simulink model "SF018A_EotProtn"  (R2013b)
settings: Solver=FixedStepDiscrete  SolverMode=SingleTasking  StartTime=0.0  StopTime=0.002  FixedStep=.002  RelTol=1e-3
undefined symbols (not defined in the file): ALLSPDDAMPG_CNT_U08, ALLSPDGAIN_CNT_U08, ARCHGLBPRM_2MILLISEC_SEC_F32, DISTLPFILFRQ_HZ_F32, EOTDAMPGLOLIM_MOTNWTMTR_F32, EOTGAINHILIM_ULS_F32, EotProtnActvRegnBypMaxThd, EotProtnDampgSlew, EotProtnDampgVehSpdTbl, EotProtnDeltaTqThd, EotProtnDftPosn, EotProtnEntrGainVehSpdTbl, EotProtnEntrGainX, EotProtnEntrStLpFilFrq, EotProtnExitDampgY, EotProtnExitStLpFilFrq, EotProtnHwAgGain, EotProtnHwAgMax, EotProtnHwAgMin, EotProtnHwDegDampgX, EotProtnMotSpdIncptSca, EotProtnMotSpdIncptX, EotProtnMotSpdIncptY, EotProtnMotVelGain, EotProtnNormDampgY, EotProtnPosnRampStep, EotProtnRackTrvlLimrAuthyThd, EotProtnRackTrvlLimrAuthyThdLimd, EotProtnRackTrvlLimrEna, EotProtnRackTrvlLimrRng, EotProtnRackTrvlLimrRngLimd, EotProtnRackTrvlLimrVehSpdThd, EotProtnRunEotVelImpctAndSoftEndStop, EotProtnSoftEndStopAuthyThd, EotProtnSoftEndStopEna, EotProtnSoftEndStopVehSpdThd, FIRSTPTDAMPG_CNT_U08, LASTPTGAIN_CNT_U08, SOFTENDSTOPSTDI_CNT_U08, SOFTENDSTOPSTENTR_CNT_U08, SOFTENDSTOPSTEXIT_CNT_U08, SOFTENDSTOPSTNORM_CNT_U08, SYSGLBPRM_MOTTQCMDHILIM_MOTNWTMTR_F32, ZEROMOTTQCMD_MOTNWTMTR_F32
libraries: NxtrAbslt x16, FloatToFixd x14, FixdToFloat x6, Fil x5, NxtrLim x5, simulink x4, NxtrMax x4, LnrIntrpnDyn x3, NxtrSign x2, BilnrIntrpnMplXDyn x2, BilnrIntrpnMplX x1, LnrIntrpn x1
(part 3 of 5)

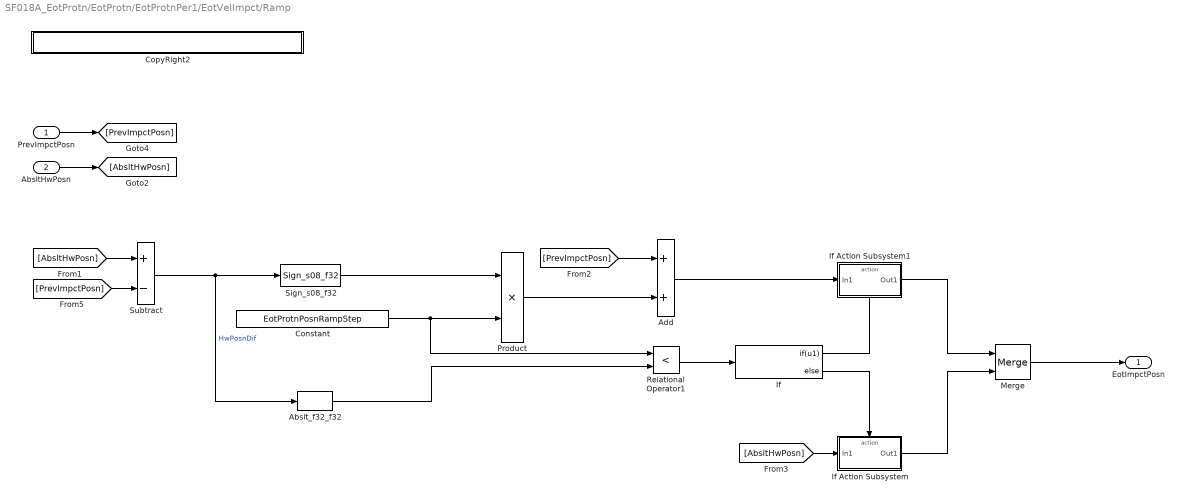
== system SF018A_EotProtn/EotProtn/EotProtnPer1/EotVelImpct/Ramp ==
  PrevImpctPosn : Inport
  AbsltHwPosn : Inport  Port=2
  Abslt_f32_f32 : NxtrAbslt/Abslt_f32_f32  RequirementInfo={'linktype_rmi_doors' '0000ba56 (/E-STEER Core/SubSystem Specifications/Application Functions/SF018A End-of-Travel Actuator Management- EOT Impact and Soft Stops)' '#SF018A_99' 'true' 'REQ: SF018A_99' '' } %GIDa_1abceffa_5429_43f7_acf2_7bb66654749d  SFunctionSpec=single y1 = Abslt_f32_f32(single u1)
      settings: AttributesFormatString=%<Name>
  Add : Sum  RequirementInfo={'linktype_rmi_doors' '0000ba56 (/E-STEER Core/SubSystem Specifications/Application Functions/SF018A End-of-Travel Actuator Management- EOT Impact and Soft Stops)' '#SF018A_99' 'true' 'REQ: SF018A_99' '' } %GIDa_4b3b0817_279b_45d5_a7ff_759bd2d41568
  Constant : Constant  RequirementInfo={'linktype_rmi_doors' '0000ba56 (/E-STEER Core/SubSystem Specifications/Application Functions/SF018A End-of-Travel Actuator Management- EOT Impact and Soft Stops)' '#SF018A_99' 'true' 'REQ: SF018A_99' '' } %GIDa_f7bca0cc_e413_4645_ac8d_d71262a020ac  Value=EotProtnPosnRampStep
  CopyRight2 : Subsystem  Description=|  mask(Copyright Information){none=on}
      | Copyright info block.                                               
      |                                                                     
      | Place copyright information at the top of every subsystem in design.
      mask prompts: none "No parameters"
      mask help: Place copyright information at the top of every subsystem in design.
      mask Display:
      | NxtrConf = 'Nexteer Confidential';
      | 
      | sys = bdroot; %handle for the current model ("system")
      | first = get_param(sys,'Created');
      | if(isempty(first))
      |     first = datestr(now,'yyyy');
      | else
      |     first = first(end-3:end);  %year is last four digits
      | end
      | 
      | last = get_param(sys,'LastModifiedDate');
      | if isempty(last)
      |     last = datestr(now,'yyyy');
      | else
      |     last = last(end-3:end);
      | end
      | 
      | if strcmp(first,last)
      |     fprintf('%s -- Copyright %s Nexteer',NxtrConf,first)
      | else
      |     fprintf('%s -- %s%s- %s Nexteer',NxtrConf,char(169),first,last)
      | end
  If : If  RequirementInfo={'linktype_rmi_doors' '0000ba56 (/E-STEER Core/SubSystem Specifications/Application Functions/SF018A End-of-Travel Actuator Management- EOT Impact and Soft Stops)' '#SF018A_99' 'true' 'REQ: SF018A_99' '' } %GIDa_742bd3cd_f3a7_4580_9ac8_68cba2588316  IfExpression=u1
  If Action Subsystem : Subsystem  RequirementInfo={'linktype_rmi_doors' '0000ba56 (/E-STEER Core/SubSystem Specifications/Application Functions/SF018A End-of-Travel Actuator Management- EOT Impact and Soft Stops)' '#SF018A_99' 'true' 'REQ: SF018A_99' '' } %GIDa_43f6df8e_6398_4b56_9d96_dcc88b087a3b  TreatAsAtomicUnit=on
  If Action Subsystem1 : Subsystem  RequirementInfo={'linktype_rmi_doors' '0000ba56 (/E-STEER Core/SubSystem Specifications/Application Functions/SF018A End-of-Travel Actuator Management- EOT Impact and Soft Stops)' '#SF018A_99' 'true' 'REQ: SF018A_99' '' } %GIDa_60fb960e_afb5_4503_a9d1_873d957e00f4  TreatAsAtomicUnit=on
  Merge : Merge  RequirementInfo={'linktype_rmi_doors' '0000ba56 (/E-STEER Core/SubSystem Specifications/Application Functions/SF018A End-of-Travel Actuator Management- EOT Impact and Soft Stops)' '#SF018A_99' 'true' 'REQ: SF018A_99' '' } %GIDa_980ed3f9_6cab_48af_a5f8_074a3afd95c0
  Product : Product  RequirementInfo={'linktype_rmi_doors' '0000ba56 (/E-STEER Core/SubSystem Specifications/Application Functions/SF018A End-of-Travel Actuator Management- EOT Impact and Soft Stops)' '#SF018A_99' 'true' 'REQ: SF018A_99' '' } %GIDa_1965b7b1_3372_4a34_81de_e822cfa0f36c  RndMeth=Zero
  Relational Operator1 : RelationalOperator  RequirementInfo={'linktype_rmi_doors' '0000ba56 (/E-STEER Core/SubSystem Specifications/Application Functions/SF018A End-of-Travel Actuator Management- EOT Impact and Soft Stops)' '#SF018A_99' 'true' 'REQ: SF018A_99' '' } %GIDa_2c3f3792_848e_4354_937e_e14b12a6658e  Operator=<  OutDataTypeStr=boolean
  Sign_s08_f32 : NxtrSign/Sign_s08_f32  RequirementInfo={'linktype_rmi_doors' '0000ba56 (/E-STEER Core/SubSystem Specifications/Application Functions/SF018A End-of-Travel Actuator Management- EOT Impact and Soft Stops)' '#SF018A_99' 'true' 'REQ: SF018A_99' '' } %GIDa_dea15310_ec68_42a1_8b11_5567d207a828  SFunctionSpec=int8 y1 = Sign_s08_f32(single u1)
  Subtract : Sum  RequirementInfo={'linktype_rmi_doors' '0000ba56 (/E-STEER Core/SubSystem Specifications/Application Functions/SF018A End-of-Travel Actuator Management- EOT Impact and Soft Stops)' '#SF018A_99' 'true' 'REQ: SF018A_99' '' } %GIDa_d23a2f2b_f22f_4421_a8b2_6f0d87dd44f6  Inputs=+-
  EotImpctPosn : Outport
  wires:
  Relational Operator1/1 -> If/1
  If/1 -> If Action Subsystem1/Action
  If/2 -> If Action Subsystem/Action
  If Action Subsystem/1(Out1) -> Merge/2
  If Action Subsystem1/1(Out1) -> Merge/1
  Add/1 -> If Action Subsystem1/1(In1)
  [AbsltHwPosn] -> If Action Subsystem/1(In1)
  Merge/1 -> EotImpctPosn/1
  [PrevImpctPosn] -> Add/1
  Product/1 -> Add/2
  Abslt_f32_f32/1 -> Relational Operator1/2
  Sign_s08_f32/1 -> Product/1
  Constant/1 -> Product/2, Relational Operator1/1
  Subtract/1 -> Sign_s08_f32/1, Abslt_f32_f32/1  "HwPosnDif"
  [PrevImpctPosn] -> Subtract/2
  [AbsltHwPosn] -> Subtract/1
  AbsltHwPosn/1 -> [AbsltHwPosn]
  PrevImpctPosn/1 -> [PrevImpctPosn]

== system SF018A_EotProtn/EotProtn/EotProtnPer1/If Action Subsystem/CopyRight2 ==

== system SF018A_EotProtn/EotProtn/EotProtnPer1/If Action Subsystem5/CopyRight2 ==

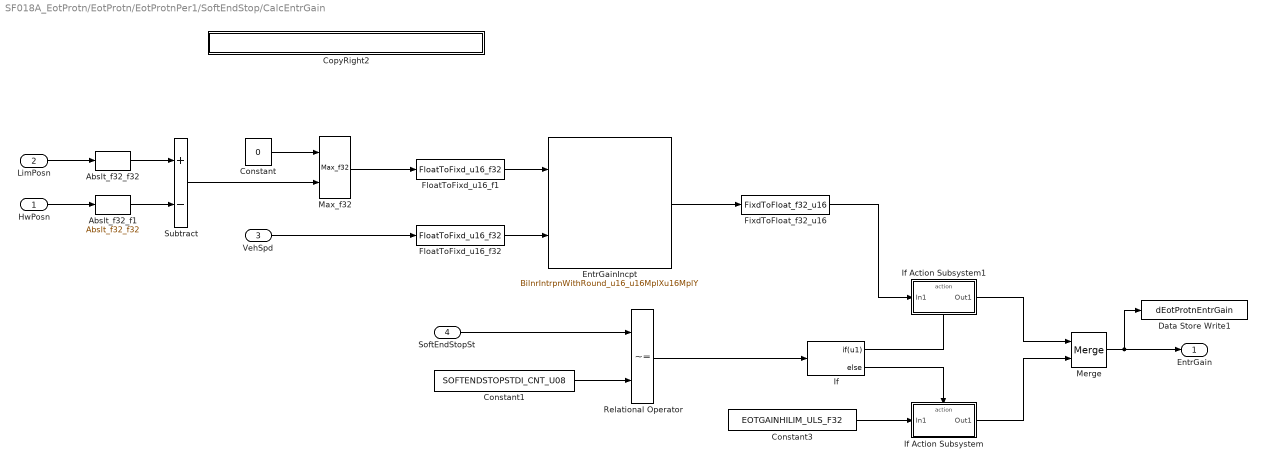
== system SF018A_EotProtn/EotProtn/EotProtnPer1/SoftEndStop/CalcEntrGain ==
  HwPosn : Inport
  LimPosn : Inport  Port=2
  VehSpd : Inport  Port=3
  SoftEndStopSt : Inport  Port=4
  Abslt_f32_f1 : NxtrAbslt/Abslt_f32_f32  SFunctionSpec=single y1 = Abslt_f32_f32(single u1)
      settings: AttributesFormatString=%<Name>
  Abslt_f32_f32 : NxtrAbslt/Abslt_f32_f32  SFunctionSpec=single y1 = Abslt_f32_f32(single u1)
      settings: AttributesFormatString=%<Name>
  Constant : Constant  Value=0  OutDataTypeStr=single
  Constant1 : Constant  Value=SOFTENDSTOPSTDI_CNT_U08
  Constant3 : Constant  RequirementInfo={'linktype_rmi_doors' '0000ba56 (/E-STEER Core/SubSystem Specifications/Application Functions/SF018A End-of-Travel Actuator Management- EOT Impact and Soft Stops)' '#SF018A_110' 'true' 'REQ: SF018A_110' '' } %GIDa_44744990_5e4e_4c9c_97f2_54307b70273a  Value=EOTGAINHILIM_ULS_F32
  CopyRight2 : Subsystem  Description=|  mask(Copyright Information){none=on}
      | Copyright info block.                                               
      |                                                                     
      | Place copyright information at the top of every subsystem in design.
      mask prompts: none "No parameters"
      mask help: Place copyright information at the top of every subsystem in design.
      mask Display:
      | NxtrConf = 'Nexteer Confidential';
      | 
      | sys = bdroot; %handle for the current model ("system")
      | first = get_param(sys,'Created');
      | if(isempty(first))
      |     first = datestr(now,'yyyy');
      | else
      |     first = first(end-3:end);  %year is last four digits
      | end
      | 
      | last = get_param(sys,'LastModifiedDate');
      | if isempty(last)
      |     last = datestr(now,'yyyy');
      | else
      |     last = last(end-3:end);
      | end
      | 
      | if strcmp(first,last)
      |     fprintf('%s -- Copyright %s Nexteer',NxtrConf,first)
      | else
      |     fprintf('%s -- %s%s- %s Nexteer',NxtrConf,char(169),first,last)
      | end
  Data Store Write1 : DataStoreWrite  DataStoreName=dEotProtnEntrGain
  EntrGainIncpt : BilnrIntrpnMplX/BilnrIntrpnWithRound_u16_u16MplXu16MplY  RequirementInfo={'linktype_rmi_doors' '0000ba56 (/E-STEER Core/SubSystem Specifications/Application Functions/SF018A End-of-Travel Actuator Management- EOT Impact and Soft Stops)' '#SF018A_106' 'true' 'REQ: SF018A_106' '' } %GIDa_4fff3482_45f7_455a_b7ca_7ca531bddd7e  MplXTbl=EotProtnEntrGainX  MplYTbl=EotProtnEntrGainY  BilnrSelnTbl=EotProtnEntrGainVehSpdTbl
      settings: AttributesFormatString=Bilnr ( u16MplX , u16MplY )
  FixdToFloat_f32_u16 : FixdToFloat/FixdToFloat_f32_u16  Param1=15
  FloatToFixd_u16_f1 : FloatToFixd/FloatToFixd_u16_f32  Param1=4
  FloatToFixd_u16_f32 : FloatToFixd/FloatToFixd_u16_f32  Param1=7
  If : If  RequirementInfo={'linktype_rmi_doors' '0000ba56 (/E-STEER Core/SubSystem Specifications/Application Functions/SF018A End-of-Travel Actuator Management- EOT Impact and Soft Stops)' '#SF018A_110' 'true' 'REQ: SF018A_110' '' } %GIDa_9ba4167e_05f8_43ad_8506_1cfb529838b9  IfExpression=u1
  If Action Subsystem : Subsystem  RequirementInfo={'linktype_rmi_doors' '0000ba56 (/E-STEER Core/SubSystem Specifications/Application Functions/SF018A End-of-Travel Actuator Management- EOT Impact and Soft Stops)' '#SF018A_110' 'true' 'REQ: SF018A_110' '' } %GIDa_2636f089_91d8_4ceb_8b94_5c1d30901327  TreatAsAtomicUnit=on
  If Action Subsystem1 : Subsystem  RequirementInfo={'linktype_rmi_doors' '0000ba56 (/E-STEER Core/SubSystem Specifications/Application Functions/SF018A End-of-Travel Actuator Management- EOT Impact and Soft Stops)' '#SF018A_110' 'true' 'REQ: SF018A_110' '' } %GIDa_4dab6c91_13d9_4980_84a7_ab8b61b230ac  TreatAsAtomicUnit=on
  Max_f32 : NxtrMax/Max_f32  SFunctionSpec=single y1 = Max_f32(single u1, single u2)
      settings: AttributesFormatString=%<Name>
  Merge : Merge  RequirementInfo={'linktype_rmi_doors' '0000ba56 (/E-STEER Core/SubSystem Specifications/Application Functions/SF018A End-of-Travel Actuator Management- EOT Impact and Soft Stops)' '#SF018A_110' 'true' 'REQ: SF018A_110' '' } %GIDa_f387e512_66e3_47bc_bfbf_7513709a11a9
  Relational Operator : RelationalOperator  RequirementInfo={'linktype_rmi_doors' '0000ba56 (/E-STEER Core/SubSystem Specifications/Application Functions/SF018A End-of-Travel Actuator Management- EOT Impact and Soft Stops)' '#SF018A_110' 'true' 'REQ: SF018A_110' '' } %GIDa_a3a9fdec_6549_4f75_9399_aedfe2c4c451  Operator=~=  OutDataTypeStr=boolean
  Subtract : Sum  RequirementInfo={'linktype_rmi_doors' '0000ba56 (/E-STEER Core/SubSystem Specifications/Application Functions/SF018A End-of-Travel Actuator Management- EOT Impact and Soft Stops)' '#SF018A_106' 'true' 'REQ: SF018A_106' '' } %GIDa_7ecf2b4b_fe31_40cc_9806_1ed7231da289  Inputs=+-
  EntrGain : Outport
  wires:
  EntrGainIncpt/1 -> FixdToFloat_f32_u16/1
  FloatToFixd_u16_f1/1 -> EntrGainIncpt/1
  Relational Operator/1 -> If/1
  FixdToFloat_f32_u16/1 -> If Action Subsystem1/1(In1)
  Max_f32/1 -> FloatToFixd_u16_f1/1
  Constant/1 -> Max_f32/1
  Constant1/1 -> Relational Operator/2
  Merge/1 -> EntrGain/1, Data Store Write1/1
  Constant3/1 -> If Action Subsystem/1(In1)
  SoftEndStopSt/1 -> Relational Operator/1
  If/1 -> If Action Subsystem1/Action
  If/2 -> If Action Subsystem/Action
  If Action Subsystem/1(Out1) -> Merge/2
  If Action Subsystem1/1(Out1) -> Merge/1
  FloatToFixd_u16_f32/1 -> EntrGainIncpt/2
  VehSpd/1 -> FloatToFixd_u16_f32/1
  Subtract/1 -> Max_f32/2
  Abslt_f32_f1/1 -> Subtract/2
  Abslt_f32_f32/1 -> Subtract/1
  LimPosn/1 -> Abslt_f32_f32/1
  HwPosn/1 -> Abslt_f32_f1/1

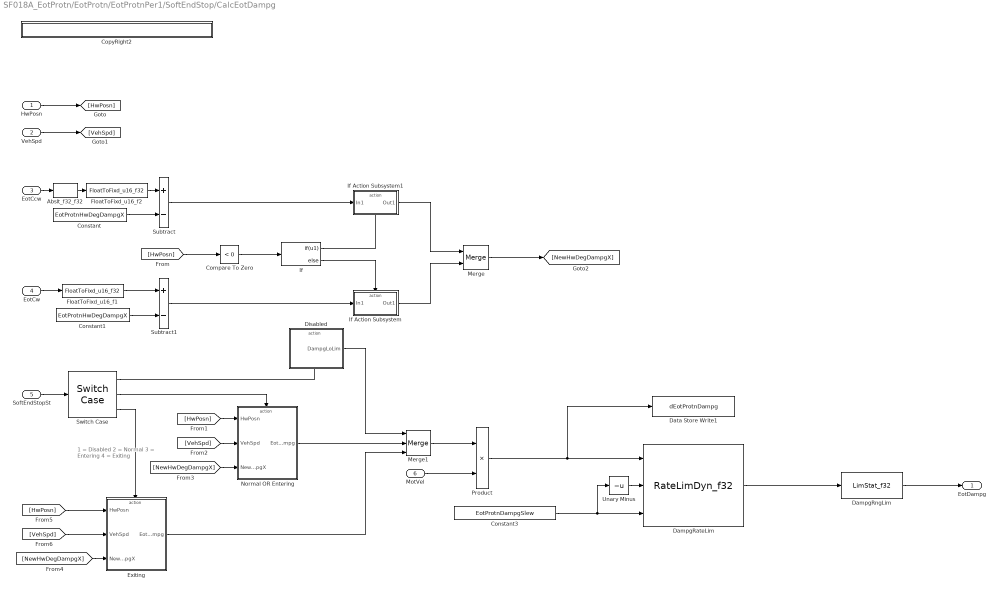
== system SF018A_EotProtn/EotProtn/EotProtnPer1/SoftEndStop/CalcEotDampg ==
  note: 1 = Disabled
      | 2 = Normal
      | 3 = Entering
      | 4 = Exiting
  HwPosn : Inport
  VehSpd : Inport  Port=2
  EotCcw : Inport  Port=3
  EotCw : Inport  Port=4
  SoftEndStopSt : Inport  Port=5
  MotVel : Inport  Port=6
  " Disabled" : Subsystem  RequirementInfo={'linktype_rmi_doors' '0000ba56 (/E-STEER Core/SubSystem Specifications/Application Functions/SF018A End-of-Travel Actuator Management- EOT Impact and Soft Stops)' '#SF018A_112' 'true' 'REQ: SF018A_112' '' } %GIDa_ecfa1b07_e2c5_474f_af19_fddfe94ef9e6
  " Exiting" : Subsystem  TreatAsAtomicUnit=on
  " Normal OR Entering" : Subsystem  TreatAsAtomicUnit=on
  Abslt_f32_f32 : NxtrAbslt/Abslt_f32_f32  SFunctionSpec=single y1 = Abslt_f32_f32(single u1)
      settings: AttributesFormatString=%<Name>
  Compare To Zero : simulink/Logic and Bit Operations/Compare To Zero  RequirementInfo={'linktype_rmi_doors' '0000ba56 (/E-STEER Core/SubSystem Specifications/Application Functions/SF018A End-of-Travel Actuator Management- EOT Impact and Soft Stops)' '#SF018A_112' 'true' 'REQ: SF018A_112' '' } %GIDa_9be31a75_f41f_436f_9025_b1c96be2af0a  relop=<  OutDataTypeStr=boolean
  Constant : Constant  RequirementInfo={'linktype_rmi_doors' '0000ba56 (/E-STEER Core/SubSystem Specifications/Application Functions/SF018A End-of-Travel Actuator Management- EOT Impact and Soft Stops)' '#SF018A_112' 'true' 'REQ: SF018A_112' '' } %GIDa_dbcb604d_2f24_40f5_8854_e760e508102d  Value=EotProtnHwDegDampgX
  Constant1 : Constant  RequirementInfo={'linktype_rmi_doors' '0000ba56 (/E-STEER Core/SubSystem Specifications/Application Functions/SF018A End-of-Travel Actuator Management- EOT Impact and Soft Stops)' '#SF018A_112' 'true' 'REQ: SF018A_112' '' } %GIDa_c66114bb_2673_4ad0_b25b_e6b85f1e3550  Value=EotProtnHwDegDampgX
  Constant3 : Constant  RequirementInfo={'linktype_rmi_doors' '0000ba56 (/E-STEER Core/SubSystem Specifications/Application Functions/SF018A End-of-Travel Actuator Management- EOT Impact and Soft Stops)' '#SF018A_107' 'true' 'REQ: SF018A_107' '' ; 'linktype_rmi_doors' '0000ba56 (/E-STEER Core/SubSystem Specifications/Application Functions/SF018A End-of-Travel Actuator Management- EOT Impact and Soft Stops)' '#SF018A_108' 'true' 'REQ: SF018A_108' '' } %GIDa_b144d1b2_0f77_499c_8b78_f2421302eedf  Value=EotProtnDampgSlew
  CopyRight2 : Subsystem  Description=|  mask(Copyright Information){none=on}
      | Copyright info block.                                               
      |                                                                     
      | Place copyright information at the top of every subsystem in design.
      mask prompts: none "No parameters"
      mask help: Place copyright information at the top of every subsystem in design.
      mask Display:
      | NxtrConf = 'Nexteer Confidential';
      | 
      | sys = bdroot; %handle for the current model ("system")
      | first = get_param(sys,'Created');
      | if(isempty(first))
      |     first = datestr(now,'yyyy');
      | else
      |     first = first(end-3:end);  %year is last four digits
      | end
      | 
      | last = get_param(sys,'LastModifiedDate');
      | if isempty(last)
      |     last = datestr(now,'yyyy');
      | else
      |     last = last(end-3:end);
      | end
      | 
      | if strcmp(first,last)
      |     fprintf('%s -- Copyright %s Nexteer',NxtrConf,first)
      | else
      |     fprintf('%s -- %s%s- %s Nexteer',NxtrConf,char(169),first,last)
      | end
  DampgRateLim : NxtrLim/RateLimDyn_f32  RequirementInfo={'linktype_rmi_doors' '0000ba56 (/E-STEER Core/SubSystem Specifications/Application Functions/SF018A End-of-Travel Actuator Management- EOT Impact and Soft Stops)' '#SF018A_107' 'true' 'REQ: SF018A_107' '' ; 'linktype_rmi_doors' '0000ba56 (/E-STEER Core/SubSystem Specifications/Application Functions/SF018A End-of-Travel Actuator Management- EOT Impact and Soft Stops)' '#SF018A_108' 'true' 'REQ: SF018A_108' '' } %GIDa_7842721c_96f0_4555_8d64_95f51b59d9d7  StVar=PrevEotDampg  Ts=ARCHGLBPRM_2MILLISEC_SEC_F32
      link override Data Store Read: DataStoreName=PrevEotDampg
      link override Data Store Write: DataStoreName=PrevEotDampg
      settings: AttributesFormatString=StVar: %<StVar>
  DampgRngLim : NxtrLim/LimStat_f32  RequirementInfo={'linktype_rmi_doors' '0000ba56 (/E-STEER Core/SubSystem Specifications/Application Functions/SF018A End-of-Travel Actuator Management- EOT Impact and Soft Stops)' '#SF018A_113' 'true' 'REQ: SF018A_113' '' } %GIDa_f21829fe_30fb_47d7_986c_fd83414cd0bc  LoLim=SYSGLBPRM_MOTTQCMDLOLIM_MOTNWTMTR_F32  HiLim=SYSGLBPRM_MOTTQCMDHILIM_MOTNWTMTR_F32
      settings: AttributesFormatString=|
      | Low Limit: %<LoLim>
      | High Limit:%<HiLim>
  Data Store Write1 : DataStoreWrite  DataStoreName=dEotProtnDampg
  FloatToFixd_u16_f1 : FloatToFixd/FloatToFixd_u16_f32  Param1=4
  FloatToFixd_u16_f2 : FloatToFixd/FloatToFixd_u16_f32  Param1=4
  If : If  RequirementInfo={'linktype_rmi_doors' '0000ba56 (/E-STEER Core/SubSystem Specifications/Application Functions/SF018A End-of-Travel Actuator Management- EOT Impact and Soft Stops)' '#SF018A_112' 'true' 'REQ: SF018A_112' '' } %GIDa_80fe16f3_461b_464d_939e_d39adab0e653  IfExpression=u1
  If Action Subsystem : Subsystem  RequirementInfo={'linktype_rmi_doors' '0000ba56 (/E-STEER Core/SubSystem Specifications/Application Functions/SF018A End-of-Travel Actuator Management- EOT Impact and Soft Stops)' '#SF018A_112' 'true' 'REQ: SF018A_112' '' } %GIDa_e943b242_c41a_47ba_8233_2176091eed70  TreatAsAtomicUnit=on
  If Action Subsystem1 : Subsystem  RequirementInfo={'linktype_rmi_doors' '0000ba56 (/E-STEER Core/SubSystem Specifications/Application Functions/SF018A End-of-Travel Actuator Management- EOT Impact and Soft Stops)' '#SF018A_112' 'true' 'REQ: SF018A_112' '' } %GIDa_bde328e5_3b39_4d8b_939f_44ff43e1078d  TreatAsAtomicUnit=on
  Merge : Merge  RequirementInfo={'linktype_rmi_doors' '0000ba56 (/E-STEER Core/SubSystem Specifications/Application Functions/SF018A End-of-Travel Actuator Management- EOT Impact and Soft Stops)' '#SF018A_112' 'true' 'REQ: SF018A_112' '' } %GIDa_c1aa902f_1f6f_4629_beda_cf4686bd9346
  Merge1 : Merge  RequirementInfo={'linktype_rmi_doors' '0000ba56 (/E-STEER Core/SubSystem Specifications/Application Functions/SF018A End-of-Travel Actuator Management- EOT Impact and Soft Stops)' '#SF018A_112' 'true' 'REQ: SF018A_112' '' } %GIDa_e0e5e6ca_8c3a_4f1c_bb6f_ec62d627a8cd  Inputs=3
  Product : Product  RequirementInfo={'linktype_rmi_doors' '0000ba56 (/E-STEER Core/SubSystem Specifications/Application Functions/SF018A End-of-Travel Actuator Management- EOT Impact and Soft Stops)' '#SF018A_112' 'true' 'REQ: SF018A_112' '' } %GIDa_edec6862_a88c_4eda_8732_0ab8679f0f39  RndMeth=Zero
  Subtract : Sum  RequirementInfo={'linktype_rmi_doors' '0000ba56 (/E-STEER Core/SubSystem Specifications/Application Functions/SF018A End-of-Travel Actuator Management- EOT Impact and Soft Stops)' '#SF018A_112' 'true' 'REQ: SF018A_112' '' } %GIDa_fd2362af_1e36_467c_917a_9f3405f6ac8b  Inputs=+-
  Subtract1 : Sum  RequirementInfo={'linktype_rmi_doors' '0000ba56 (/E-STEER Core/SubSystem Specifications/Application Functions/SF018A End-of-Travel Actuator Management- EOT Impact and Soft Stops)' '#SF018A_112' 'true' 'REQ: SF018A_112' '' } %GIDa_c20c8d7b_5540_434b_b02f_ea8a96eddc7e  Inputs=+-
  Switch Case : SwitchCase  RequirementInfo={'linktype_rmi_doors' '0000ba56 (/E-STEER Core/SubSystem Specifications/Application Functions/SF018A End-of-Travel Actuator Management- EOT Impact and Soft Stops)' '#SF018A_112' 'true' 'REQ: SF018A_112' '' } %GIDa_87bdb368_40c5_441a_b972_d5c9fc169f63  CaseConditions={1,[2,3],4}  ShowDefaultCase=off
  Unary Minus : UnaryMinus  RequirementInfo={'linktype_rmi_doors' '0000ba56 (/E-STEER Core/SubSystem Specifications/Application Functions/SF018A End-of-Travel Actuator Management- EOT Impact and Soft Stops)' '#SF018A_107' 'true' 'REQ: SF018A_107' '' ; 'linktype_rmi_doors' '0000ba56 (/E-STEER Core/SubSystem Specifications/Application Functions/SF018A End-of-Travel Actuator Management- EOT Impact and Soft Stops)' '#SF018A_108' 'true' 'REQ: SF018A_108' '' } %GIDa_64f4e9aa_203f_4d05_a587_f31f06ac7c23
  EotDampg : Outport
  wires:
  DampgRngLim/1 -> EotDampg/1
  SoftEndStopSt/1 -> Switch Case/1
  Merge1/1 -> Product/1
  DampgRateLim/1 -> DampgRngLim/1
  Subtract/1 -> If Action Subsystem1/1(In1)
  Constant/1 -> Subtract/2
  [HwPosn] -> " Normal OR Entering"/1(HwPosn)
  Unary Minus/1 -> DampgRateLim/2
  Constant3/1 -> DampgRateLim/3, Unary Minus/1
  Product/1 -> DampgRateLim/1, Data Store Write1/1
  MotVel/1 -> Product/2
  " Exiting"/1(EotDampg) -> Merge1/3
  " Normal OR Entering"/1(EotDampg) -> Merge1/2
  " Disabled"/1(DampgLoLim) -> Merge1/1
  [VehSpd] -> " Exiting"/2(VehSpd)
  [HwPosn] -> " Exiting"/1(HwPosn)
  [NewHwDegDampgX] -> " Exiting"/3(NewHwDegDampgX)
  Switch Case/3 -> " Exiting"/Action
  [VehSpd] -> " Normal OR Entering"/2(VehSpd)
  [NewHwDegDampgX] -> " Normal OR Entering"/3(NewHwDegDampgX)
  Switch Case/2 -> " Normal OR Entering"/Action
  Switch Case/1 -> " Disabled"/Action
  Merge/1 -> [NewHwDegDampgX]
  Subtract1/1 -> If Action Subsystem/1(In1)
  Compare To Zero/1 -> If/1
  If/1 -> If Action Subsystem1/Action
  If/2 -> If Action Subsystem/Action
  If Action Subsystem/1(Out1) -> Merge/2
  If Action Subsystem1/1(Out1) -> Merge/1
  Constant1/1 -> Subtract1/2
  FloatToFixd_u16_f1/1 -> Subtract1/1
  EotCw/1 -> FloatToFixd_u16_f1/1
  [HwPosn] -> Compare To Zero/1
  FloatToFixd_u16_f2/1 -> Subtract/1
  EotCcw/1 -> Abslt_f32_f32/1
  VehSpd/1 -> [VehSpd]
  HwPosn/1 -> [HwPosn]
  Abslt_f32_f32/1 -> FloatToFixd_u16_f2/1

== system SF018A_EotProtn/EotProtn/EotProtnPer1/SoftEndStop/CalcEotGain ==
  note: 1 = Disabled
      | 2 = Normal
      | 3 = Entering
      | 4 = Exiting
  EntrGain : Inport
  SoftEndStopSt : Inport  Port=2
  ExitGain : Inport  Port=3
  " Disabled" : Subsystem  RequirementInfo={'linktype_rmi_doors' '0000ba56 (/E-STEER Core/SubSystem Specifications/Application Functions/SF018A End-of-Travel Actuator Management- EOT Impact and Soft Stops)' '#SF018A_110' 'true' 'REQ: SF018A_110' '' } %GIDa_08480493_e720_439d_8401_9a38b0039812
  " Exiting" : Subsystem
  Constant : Constant  RequirementInfo={'linktype_rmi_doors' '0000ba56 (/E-STEER Core/SubSystem Specifications/Application Functions/SF018A End-of-Travel Actuator Management- EOT Impact and Soft Stops)' '#SF018A_110' 'true' 'REQ: SF018A_110' '' } %GIDa_76f8a074_7de7_475c_bca0_9f449228cd27  Value=EOTGAINHILIM_ULS_F32
  CopyRight2 : Subsystem  Description=|  mask(Copyright Information){none=on}
      | Copyright info block.                                               
      |                                                                     
      | Place copyright information at the top of every subsystem in design.
      mask prompts: none "No parameters"
      mask help: Place copyright information at the top of every subsystem in design.
      mask Display:
      | NxtrConf = 'Nexteer Confidential';
      | 
      | sys = bdroot; %handle for the current model ("system")
      | first = get_param(sys,'Created');
      | if(isempty(first))
      |     first = datestr(now,'yyyy');
      | else
      |     first = first(end-3:end);  %year is last four digits
      | end
      | 
      | last = get_param(sys,'LastModifiedDate');
      | if isempty(last)
      |     last = datestr(now,'yyyy');
      | else
      |     last = last(end-3:end);
      | end
      | 
      | if strcmp(first,last)
      |     fprintf('%s -- Copyright %s Nexteer',NxtrConf,first)
      | else
      |     fprintf('%s -- %s%s- %s Nexteer',NxtrConf,char(169),first,last)
      | end
  Data Store Write1 : DataStoreWrite  DataStoreName=dEotProtnEotGain
  Entering or Normal : Subsystem
  Merge : Merge  Inputs=3
  Switch Case : SwitchCase  CaseConditions={1,4}
  EotGain : Outport
  wires:
  SoftEndStopSt/1 -> Switch Case/1
  " Disabled"/1(Out1) -> Merge/1
  Constant/1 -> " Disabled"/1(In1)
  Merge/1 -> EotGain/1, Data Store Write1/1
  EntrGain/1 -> Entering or Normal/1(In1)
  ExitGain/1 -> " Exiting"/1(In1)
  Entering or Normal/1(Out1) -> Merge/3
  " Exiting"/1(Out1) -> Merge/2
  Switch Case/3 -> Entering or Normal/Action
  Switch Case/2 -> " Exiting"/Action
  Switch Case/1 -> " Disabled"/Action

== system SF018A_EotProtn/EotProtn/EotProtnPer1/SoftEndStop/CalcExitGain ==
  HwTq : Inport
  HwPosn : Inport  Port=2
  PrevEotAssiSca : Inport  Port=3
  Abslt_f32_f32 : NxtrAbslt/Abslt_f32_f32  SFunctionSpec=single y1 = Abslt_f32_f32(single u1)
      settings: AttributesFormatString=%<Name>
  CopyRight2 : Subsystem  Description=|  mask(Copyright Information){none=on}
      | Copyright info block.                                               
      |                                                                     
      | Place copyright information at the top of every subsystem in design.
      mask prompts: none "No parameters"
      mask help: Place copyright information at the top of every subsystem in design.
      mask Display:
      | NxtrConf = 'Nexteer Confidential';
      | 
      | sys = bdroot; %handle for the current model ("system")
      | first = get_param(sys,'Created');
      | if(isempty(first))
      |     first = datestr(now,'yyyy');
      | else
      |     first = first(end-3:end);  %year is last four digits
      | end
      | 
      | last = get_param(sys,'LastModifiedDate');
      | if isempty(last)
      |     last = datestr(now,'yyyy');
      | else
      |     last = last(end-3:end);
      | end
      | 
      | if strcmp(first,last)
      |     fprintf('%s -- Copyright %s Nexteer',NxtrConf,first)
      | else
      |     fprintf('%s -- %s%s- %s Nexteer',NxtrConf,char(169),first,last)
      | end
  Data Store Write1 : DataStoreWrite  DataStoreName=dEotProtnExitGain
  FilLpUpdOutp : Fil/FilLpUpdOutp  StVar=HwTqLpFil
      settings: AttributesFormatString=StVar: %<StVar>
  FixdToFloat_f32_u16 : FixdToFloat/FixdToFloat_f32_u16  Param1=8
  FloatToFixd_u16_f32 : FloatToFixd/FloatToFixd_u16_f32  Param1=12
  Max_f32 : NxtrMax/Max_f32  RequirementInfo={'linktype_rmi_doors' '0000ba56 (/E-STEER Core/SubSystem Specifications/Application Functions/SF018A End-of-Travel Actuator Management- EOT Impact and Soft Stops)' '#SF018A_106' 'true' 'REQ: SF018A_106' '' } %GIDa_2332db26_7b5a_450a_9ed5_06682af17ddf  SFunctionSpec=single y1 = Max_f32(single u1, single u2)
      settings: AttributesFormatString=%<Name>
  Product : Product  RndMeth=Zero
  Sign_s08_f32 : NxtrSign/Sign_s08_f32  SFunctionSpec=int8 y1 = Sign_s08_f32(single u1)
  TqGainTbl : LnrIntrpn/LnrIntrpn_u16_u16VariXu16VariY  RequirementInfo={'linktype_rmi_doors' '0000ba56 (/E-STEER Core/SubSystem Specifications/Application Functions/SF018A End-of-Travel Actuator Management- EOT Impact and Soft Stops)' '#SF018A_106' 'true' 'REQ: SF018A_106' '' } %GIDa_1f060768_d7a3_4390_b9e3_be263574284b  XTbl=EotProtnHwTqScaX  YTbl=HWTQSCAY_ULS_U8P8
      settings: AttributesFormatString=Lnr ( u16VariX , u16VariY )
  ExitGain : Outport
  FildHwTq : Outport  Port=2
  wires:
  TqGainTbl/1 -> FixdToFloat_f32_u16/1
  FilLpUpdOutp/1 -> FildHwTq/1
  Product/1 -> FilLpUpdOutp/1
  Sign_s08_f32/1 -> Product/2
  HwPosn/1 -> Sign_s08_f32/1
  Max_f32/1 -> ExitGain/1, Data Store Write1/1
  PrevEotAssiSca/1 -> Max_f32/1
  FixdToFloat_f32_u16/1 -> Max_f32/2
  FloatToFixd_u16_f32/1 -> TqGainTbl/1
  Abslt_f32_f32/1 -> FloatToFixd_u16_f32/1
  HwTq/1 -> Abslt_f32_f32/1, Product/1

== system SF018A_EotProtn/EotProtn/EotProtnPer1/SoftEndStop/CopyRight2 ==

== system SF018A_EotProtn/EotProtn/EotProtnPer1/SoftEndStop/FildEotGain ==
  note: Disabled
  note: 1 = Disabled
      | 2 = Normal
      | 3 = Entering
      | 4 = Exiting
  note: Normal or Entering
  note: Exiting
  SoftEndStopSt : Inport
  EotGain : Inport  Port=2
  Constant : Constant  RequirementInfo={'linktype_rmi_doors' '0000ba56 (/E-STEER Core/SubSystem Specifications/Application Functions/SF018A End-of-Travel Actuator Management- EOT Impact and Soft Stops)' '#SF018A_111' 'true' 'REQ: SF018A_111' '' } %GIDa_d4377fc2_35ca_45e0_9a03_090c21e250e7  Value=DISTLPFILFRQ_HZ_F32
  Constant1 : Constant  RequirementInfo={'linktype_rmi_doors' '0000ba56 (/E-STEER Core/SubSystem Specifications/Application Functions/SF018A End-of-Travel Actuator Management- EOT Impact and Soft Stops)' '#SF018A_111' 'true' 'REQ: SF018A_111' '' } %GIDa_0b223ea8_c633_48a7_9b5a_24f3a3ad4ba1  Value=EotProtnExitStLpFilFrq
  Constant2 : Constant  RequirementInfo={'linktype_rmi_doors' '0000ba56 (/E-STEER Core/SubSystem Specifications/Application Functions/SF018A End-of-Travel Actuator Management- EOT Impact and Soft Stops)' '#SF018A_111' 'true' 'REQ: SF018A_111' '' } %GIDa_b73c8a65_7c11_42d6_a57c_7756ca0741f9  Value=EotProtnEntrStLpFilFrq
  CopyRight2 : Subsystem  Description=|  mask(Copyright Information){none=on}
      | Copyright info block.                                               
      |                                                                     
      | Place copyright information at the top of every subsystem in design.
      mask prompts: none "No parameters"
      mask help: Place copyright information at the top of every subsystem in design.
      mask Display:
      | NxtrConf = 'Nexteer Confidential';
      | 
      | sys = bdroot; %handle for the current model ("system")
      | first = get_param(sys,'Created');
      | if(isempty(first))
      |     first = datestr(now,'yyyy');
      | else
      |     first = first(end-3:end);  %year is last four digits
      | end
      | 
      | last = get_param(sys,'LastModifiedDate');
      | if isempty(last)
      |     last = datestr(now,'yyyy');
      | else
      |     last = last(end-3:end);
      | end
      | 
      | if strcmp(first,last)
      |     fprintf('%s -- Copyright %s Nexteer',NxtrConf,first)
      | else
      |     fprintf('%s -- %s%s- %s Nexteer',NxtrConf,char(169),first,last)
      | end
  Data Store Write2 : DataStoreWrite  DataStoreName=dEotProtnEotAssiSca
  FilLpUpdGain : Fil/FilLpUpdGain  RequirementInfo={'linktype_rmi_doors' '0000ba56 (/E-STEER Core/SubSystem Specifications/Application Functions/SF018A End-of-Travel Actuator Management- EOT Impact and Soft Stops)' '#SF018A_111' 'true' 'REQ: SF018A_111' '' } %GIDa_868967d1_a9f8_44e4_acea_e148f2af3442  Ts=ARCHGLBPRM_2MILLISEC_SEC_F32  StVar=EotAssiScaLpFil
      settings: AttributesFormatString=|
      | Ts: %<Ts>
      | StVar: %<StVar>
  FilLpUpdOutp : Fil/FilLpUpdOutp  RequirementInfo={'linktype_rmi_doors' '0000ba56 (/E-STEER Core/SubSystem Specifications/Application Functions/SF018A End-of-Travel Actuator Management- EOT Impact and Soft Stops)' '#SF018A_111' 'true' 'REQ: SF018A_111' '' } %GIDa_b0455bb8_047c_40b1_9af4_7987ad17d570  StVar=EotAssiScaLpFil
      settings: AttributesFormatString=StVar: %<StVar>
  If Action Subsystem3 : Subsystem  RequirementInfo={'linktype_rmi_doors' '0000ba56 (/E-STEER Core/SubSystem Specifications/Application Functions/SF018A End-of-Travel Actuator Management- EOT Impact and Soft Stops)' '#SF018A_111' 'true' 'REQ: SF018A_111' '' } %GIDa_42650f4e_4948_4e8d_b4e1_7cad7c42358e  TreatAsAtomicUnit=on
  If Action Subsystem4 : Subsystem  RequirementInfo={'linktype_rmi_doors' '0000ba56 (/E-STEER Core/SubSystem Specifications/Application Functions/SF018A End-of-Travel Actuator Management- EOT Impact and Soft Stops)' '#SF018A_111' 'true' 'REQ: SF018A_111' '' } %GIDa_f251395e_b697_4d24_b216_4a4b758d11c7  TreatAsAtomicUnit=on
  If Action Subsystem5 : Subsystem  RequirementInfo={'linktype_rmi_doors' '0000ba56 (/E-STEER Core/SubSystem Specifications/Application Functions/SF018A End-of-Travel Actuator Management- EOT Impact and Soft Stops)' '#SF018A_111' 'true' 'REQ: SF018A_111' '' } %GIDa_dbd13371_202c_4a84_bb31_10f12800c8d6  TreatAsAtomicUnit=on
  Merge : Merge  RequirementInfo={'linktype_rmi_doors' '0000ba56 (/E-STEER Core/SubSystem Specifications/Application Functions/SF018A End-of-Travel Actuator Management- EOT Impact and Soft Stops)' '#SF018A_111' 'true' 'REQ: SF018A_111' '' } %GIDa_0d86ac25_4b01_4bfe_bda9_4046b346e3c4  Inputs=3
  Switch Case : SwitchCase  RequirementInfo={'linktype_rmi_doors' '0000ba56 (/E-STEER Core/SubSystem Specifications/Application Functions/SF018A End-of-Travel Actuator Management- EOT Impact and Soft Stops)' '#SF018A_111' 'true' 'REQ: SF018A_111' '' } %GIDa_42256054_e645_47ae_a552_fd5b47b732bb  CaseConditions={1,4}
  EotAssiSca : Outport
  wires:
  FilLpUpdOutp/1 -> Data Store Write2/1, EotAssiSca/1
  EotGain/1 -> FilLpUpdOutp/1
  Constant2/1 -> If Action Subsystem4/1(In1)
  Constant1/1 -> If Action Subsystem5/1(In1)
  Constant/1 -> If Action Subsystem3/1(In1)
  Switch Case/3 -> If Action Subsystem4/Action
  Switch Case/2 -> If Action Subsystem5/Action
  Switch Case/1 -> If Action Subsystem3/Action
  SoftEndStopSt/1 -> Switch Case/1
  If Action Subsystem3/1(Out1) -> Merge/1
  If Action Subsystem5/1(Out1) -> Merge/2
  If Action Subsystem4/1(Out1) -> Merge/3
  Merge/1 -> FilLpUpdGain/1

== system SF018A_EotProtn/EotProtn/EotProtnPer1/SoftEndStop/If Action Subsystem2 ==
  In1 : Inport
  Action Port : ActionPort  ActionType=else
  CopyRight2 : Subsystem  Description=|  mask(Copyright Information){none=on}
      | Copyright info block.                                               
      |                                                                     
      | Place copyright information at the top of every subsystem in design.
      mask prompts: none "No parameters"
      mask help: Place copyright information at the top of every subsystem in design.
      mask Display:
      | NxtrConf = 'Nexteer Confidential';
      | 
      | sys = bdroot; %handle for the current model ("system")
      | first = get_param(sys,'Created');
      | if(isempty(first))
      |     first = datestr(now,'yyyy');
      | else
      |     first = first(end-3:end);  %year is last four digits
      | end
      | 
      | last = get_param(sys,'LastModifiedDate');
      | if isempty(last)
      |     last = datestr(now,'yyyy');
      | else
      |     last = last(end-3:end);
      | end
      | 
      | if strcmp(first,last)
      |     fprintf('%s -- Copyright %s Nexteer',NxtrConf,first)
      | else
      |     fprintf('%s -- %s%s- %s Nexteer',NxtrConf,char(169),first,last)
      | end
  Out1 : Outport
  wires:
  In1/1 -> Out1/1

== system SF018A_EotProtn/EotProtn/EotProtnPer1/SoftEndStop/If Action Subsystem4 ==
  In1 : Inport
  Action Port : ActionPort  ActionType=then
  CopyRight2 : Subsystem  Description=|  mask(Copyright Information){none=on}
      | Copyright info block.                                               
      |                                                                     
      | Place copyright information at the top of every subsystem in design.
      mask prompts: none "No parameters"
      mask help: Place copyright information at the top of every subsystem in design.
      mask Display:
      | NxtrConf = 'Nexteer Confidential';
      | 
      | sys = bdroot; %handle for the current model ("system")
      | first = get_param(sys,'Created');
      | if(isempty(first))
      |     first = datestr(now,'yyyy');
      | else
      |     first = first(end-3:end);  %year is last four digits
      | end
      | 
      | last = get_param(sys,'LastModifiedDate');
      | if isempty(last)
      |     last = datestr(now,'yyyy');
      | else
      |     last = last(end-3:end);
      | end
      | 
      | if strcmp(first,last)
      |     fprintf('%s -- Copyright %s Nexteer',NxtrConf,first)
      | else
      |     fprintf('%s -- %s%s- %s Nexteer',NxtrConf,char(169),first,last)
      | end
  Out1 : Outport
  wires:
  In1/1 -> Out1/1

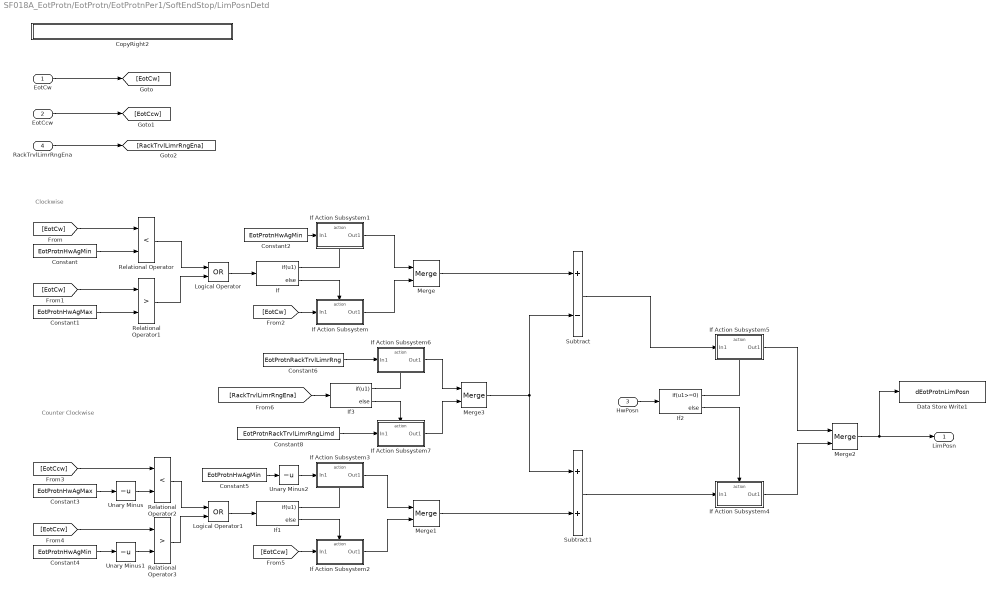
== system SF018A_EotProtn/EotProtn/EotProtnPer1/SoftEndStop/LimPosnDetd ==
  note: Clockwise
  note: Counter Clockwise
  EotCw : Inport
  EotCcw : Inport  Port=2
  HwPosn : Inport  Port=3
  RackTrvlLimrRngEna : Inport  Port=4
  Constant : Constant  RequirementInfo={'linktype_rmi_doors' '0000ba56 (/E-STEER Core/SubSystem Specifications/Application Functions/SF018A End-of-Travel Actuator Management- EOT Impact and Soft Stops)' '#SF018A_169' 'true' 'REQ: SF018A_169' '' } %GIDa_6e994ea3_46fd_4b31_bead_737a86c0690f  Value=EotProtnHwAgMin
  Constant1 : Constant  RequirementInfo={'linktype_rmi_doors' '0000ba56 (/E-STEER Core/SubSystem Specifications/Application Functions/SF018A End-of-Travel Actuator Management- EOT Impact and Soft Stops)' '#SF018A_169' 'true' 'REQ: SF018A_169' '' } %GIDa_115d3871_fa7c_4292_8e50_3386b9c580db  Value=EotProtnHwAgMax
  Constant2 : Constant  RequirementInfo={'linktype_rmi_doors' '0000ba56 (/E-STEER Core/SubSystem Specifications/Application Functions/SF018A End-of-Travel Actuator Management- EOT Impact and Soft Stops)' '#SF018A_169' 'true' 'REQ: SF018A_169' '' } %GIDa_154df6a6_622f_4ce5_9dbd_29cb8f6fa1fe  Value=EotProtnHwAgMin
  Constant3 : Constant  RequirementInfo={'linktype_rmi_doors' '0000ba56 (/E-STEER Core/SubSystem Specifications/Application Functions/SF018A End-of-Travel Actuator Management- EOT Impact and Soft Stops)' '#SF018A_169' 'true' 'REQ: SF018A_169' '' } %GIDa_dc4d9de5_8969_4d64_8a61_d25289d3986f  Value=EotProtnHwAgMax
  Constant4 : Constant  RequirementInfo={'linktype_rmi_doors' '0000ba56 (/E-STEER Core/SubSystem Specifications/Application Functions/SF018A End-of-Travel Actuator Management- EOT Impact and Soft Stops)' '#SF018A_169' 'true' 'REQ: SF018A_169' '' } %GIDa_2618cca3_834d_45ba_b0ae_a572b07e770b  Value=EotProtnHwAgMin
  Constant5 : Constant  RequirementInfo={'linktype_rmi_doors' '0000ba56 (/E-STEER Core/SubSystem Specifications/Application Functions/SF018A End-of-Travel Actuator Management- EOT Impact and Soft Stops)' '#SF018A_169' 'true' 'REQ: SF018A_169' '' } %GIDa_35fc3b1b_cb73_4c11_b5ca_9791005708bd  Value=EotProtnHwAgMin
  Constant6 : Constant  RequirementInfo={'linktype_rmi_doors' '0000ba56 (/E-STEER Core/SubSystem Specifications/Application Functions/SF018A End-of-Travel Actuator Management- EOT Impact and Soft Stops)' '#SF018A_171' 'true' 'REQ: SF018A_171' '' } %GIDa_9f0d44a5_b1b7_418c_8ccf_b55d0ba21366  Value=EotProtnRackTrvlLimrRng
  Constant8 : Constant  RequirementInfo={'linktype_rmi_doors' '0000ba56 (/E-STEER Core/SubSystem Specifications/Application Functions/SF018A End-of-Travel Actuator Management- EOT Impact and Soft Stops)' '#SF018A_171' 'true' 'REQ: SF018A_171' '' } %GIDa_dff964e5_4670_4efa_8fea_c4c2b40ceef6  Value=EotProtnRackTrvlLimrRngLimd
  CopyRight2 : Subsystem  Description=|  mask(Copyright Information){none=on}
      | Copyright info block.                                               
      |                                                                     
      | Place copyright information at the top of every subsystem in design.
      mask prompts: none "No parameters"
      mask help: Place copyright information at the top of every subsystem in design.
      mask Display:
      | NxtrConf = 'Nexteer Confidential';
      | 
      | sys = bdroot; %handle for the current model ("system")
      | first = get_param(sys,'Created');
      | if(isempty(first))
      |     first = datestr(now,'yyyy');
      | else
      |     first = first(end-3:end);  %year is last four digits
      | end
      | 
      | last = get_param(sys,'LastModifiedDate');
      | if isempty(last)
      |     last = datestr(now,'yyyy');
      | else
      |     last = last(end-3:end);
      | end
      | 
      | if strcmp(first,last)
      |     fprintf('%s -- Copyright %s Nexteer',NxtrConf,first)
      | else
      |     fprintf('%s -- %s%s- %s Nexteer',NxtrConf,char(169),first,last)
      | end
  Data Store Write1 : DataStoreWrite  DataStoreName=dEotProtnLimPosn
  If : If  RequirementInfo={'linktype_rmi_doors' '0000ba56 (/E-STEER Core/SubSystem Specifications/Application Functions/SF018A End-of-Travel Actuator Management- EOT Impact and Soft Stops)' '#SF018A_169' 'true' 'REQ: SF018A_169' '' } %GIDa_1d4f653e_51dc_4363_8e11_0b145b84baa1  IfExpression=u1
  If Action Subsystem : Subsystem  RequirementInfo={'linktype_rmi_doors' '0000ba56 (/E-STEER Core/SubSystem Specifications/Application Functions/SF018A End-of-Travel Actuator Management- EOT Impact and Soft Stops)' '#SF018A_169' 'true' 'REQ: SF018A_169' '' } %GIDa_6f02711a_cba5_4424_b99d_a805674f91c0  TreatAsAtomicUnit=on
  If Action Subsystem1 : Subsystem  RequirementInfo={'linktype_rmi_doors' '0000ba56 (/E-STEER Core/SubSystem Specifications/Application Functions/SF018A End-of-Travel Actuator Management- EOT Impact and Soft Stops)' '#SF018A_169' 'true' 'REQ: SF018A_169' '' } %GIDa_da5c21bb_332f_4aa2_ba23_e492b5ac0de2  TreatAsAtomicUnit=on
  If Action Subsystem2 : Subsystem  RequirementInfo={'linktype_rmi_doors' '0000ba56 (/E-STEER Core/SubSystem Specifications/Application Functions/SF018A End-of-Travel Actuator Management- EOT Impact and Soft Stops)' '#SF018A_169' 'true' 'REQ: SF018A_169' '' } %GIDa_af13da07_8d6d_4c29_8a66_b94238018384  TreatAsAtomicUnit=on
  If Action Subsystem3 : Subsystem  RequirementInfo={'linktype_rmi_doors' '0000ba56 (/E-STEER Core/SubSystem Specifications/Application Functions/SF018A End-of-Travel Actuator Management- EOT Impact and Soft Stops)' '#SF018A_169' 'true' 'REQ: SF018A_169' '' } %GIDa_cd9406fd_ad9c_4fe2_8f01_e79ca9da919f  TreatAsAtomicUnit=on
  If Action Subsystem4 : Subsystem  TreatAsAtomicUnit=on
  If Action Subsystem5 : Subsystem  TreatAsAtomicUnit=on
  If Action Subsystem6 : Subsystem  RequirementInfo={'linktype_rmi_doors' '0000ba56 (/E-STEER Core/SubSystem Specifications/Application Functions/SF018A End-of-Travel Actuator Management- EOT Impact and Soft Stops)' '#SF018A_171' 'true' 'REQ: SF018A_171' '' } %GIDa_39a4751f_a904_4d72_b65a_30f9b18f41e5  TreatAsAtomicUnit=on
  If Action Subsystem7 : Subsystem  RequirementInfo={'linktype_rmi_doors' '0000ba56 (/E-STEER Core/SubSystem Specifications/Application Functions/SF018A End-of-Travel Actuator Management- EOT Impact and Soft Stops)' '#SF018A_171' 'true' 'REQ: SF018A_171' '' } %GIDa_4c4949fc_c9d5_494d_8805_2521382ce9f9  TreatAsAtomicUnit=on
  If1 : If  RequirementInfo={'linktype_rmi_doors' '0000ba56 (/E-STEER Core/SubSystem Specifications/Application Functions/SF018A End-of-Travel Actuator Management- EOT Impact and Soft Stops)' '#SF018A_169' 'true' 'REQ: SF018A_169' '' } %GIDa_0b4cf865_fc9d_4eb6_97c7_0946a2aa4fb2  IfExpression=u1
  If2 : If  IfExpression=u1>=0
  If3 : If  RequirementInfo={'linktype_rmi_doors' '0000ba56 (/E-STEER Core/SubSystem Specifications/Application Functions/SF018A End-of-Travel Actuator Management- EOT Impact and Soft Stops)' '#SF018A_171' 'true' 'REQ: SF018A_171' '' } %GIDa_9123ce21_2e1c_4700_81ee_60eaf73af501  IfExpression=u1
  Logical Operator : Logic  RequirementInfo={'linktype_rmi_doors' '0000ba56 (/E-STEER Core/SubSystem Specifications/Application Functions/SF018A End-of-Travel Actuator Management- EOT Impact and Soft Stops)' '#SF018A_169' 'true' 'REQ: SF018A_169' '' } %GIDa_c3a273c9_0440_45d4_887c_1d301a03f322  Operator=OR  AllPortsSameDT=off  OutDataTypeStr=boolean
  Logical Operator1 : Logic  RequirementInfo={'linktype_rmi_doors' '0000ba56 (/E-STEER Core/SubSystem Specifications/Application Functions/SF018A End-of-Travel Actuator Management- EOT Impact and Soft Stops)' '#SF018A_169' 'true' 'REQ: SF018A_169' '' } %GIDa_72d911b1_b185_474c_9ea6_b9b0acf8246b  Operator=OR  AllPortsSameDT=off  OutDataTypeStr=boolean
  Merge : Merge  RequirementInfo={'linktype_rmi_doors' '0000ba56 (/E-STEER Core/SubSystem Specifications/Application Functions/SF018A End-of-Travel Actuator Management- EOT Impact and Soft Stops)' '#SF018A_169' 'true' 'REQ: SF018A_169' '' } %GIDa_68190868_7aa2_483a_bd88_19b4fd7775ef
  Merge1 : Merge  RequirementInfo={'linktype_rmi_doors' '0000ba56 (/E-STEER Core/SubSystem Specifications/Application Functions/SF018A End-of-Travel Actuator Management- EOT Impact and Soft Stops)' '#SF018A_169' 'true' 'REQ: SF018A_169' '' } %GIDa_7dc9374b_a207_4ee1_b50e_6f2b5bce6f84
  Merge2 : Merge
  Merge3 : Merge  RequirementInfo={'linktype_rmi_doors' '0000ba56 (/E-STEER Core/SubSystem Specifications/Application Functions/SF018A End-of-Travel Actuator Management- EOT Impact and Soft Stops)' '#SF018A_171' 'true' 'REQ: SF018A_171' '' } %GIDa_b2c9b1da_5f0b_4acc_9f73_84d9d4a81e0e
  Relational Operator : RelationalOperator  RequirementInfo={'linktype_rmi_doors' '0000ba56 (/E-STEER Core/SubSystem Specifications/Application Functions/SF018A End-of-Travel Actuator Management- EOT Impact and Soft Stops)' '#SF018A_169' 'true' 'REQ: SF018A_169' '' } %GIDa_badd5817_b2c3_43ef_a3e7_fc513af5252a  Operator=<  OutDataTypeStr=boolean
  Relational Operator1 : RelationalOperator  RequirementInfo={'linktype_rmi_doors' '0000ba56 (/E-STEER Core/SubSystem Specifications/Application Functions/SF018A End-of-Travel Actuator Management- EOT Impact and Soft Stops)' '#SF018A_169' 'true' 'REQ: SF018A_169' '' } %GIDa_12c9aacf_2d4b_413e_8b11_17ad13402905  Operator=>  OutDataTypeStr=boolean
  Relational Operator2 : RelationalOperator  RequirementInfo={'linktype_rmi_doors' '0000ba56 (/E-STEER Core/SubSystem Specifications/Application Functions/SF018A End-of-Travel Actuator Management- EOT Impact and Soft Stops)' '#SF018A_169' 'true' 'REQ: SF018A_169' '' } %GIDa_8b4f1609_2c6f_4133_a056_c6b6d52f5640  Operator=<  OutDataTypeStr=boolean
  Relational Operator3 : RelationalOperator  RequirementInfo={'linktype_rmi_doors' '0000ba56 (/E-STEER Core/SubSystem Specifications/Application Functions/SF018A End-of-Travel Actuator Management- EOT Impact and Soft Stops)' '#SF018A_169' 'true' 'REQ: SF018A_169' '' } %GIDa_19bd66cf_ec70_4def_9785_0932e01a9739  Operator=>  OutDataTypeStr=boolean
  Subtract : Sum  RequirementInfo={'linktype_rmi_doors' '0000ba56 (/E-STEER Core/SubSystem Specifications/Application Functions/SF018A End-of-Travel Actuator Management- EOT Impact and Soft Stops)' '#SF018A_170' 'true' 'REQ: SF018A_170' '' } %GIDa_7e9a77ef_5b7d_4fdd_b0f9_581fe78811e1  Inputs=+-
  Subtract1 : Sum  RequirementInfo={'linktype_rmi_doors' '0000ba56 (/E-STEER Core/SubSystem Specifications/Application Functions/SF018A End-of-Travel Actuator Management- EOT Impact and Soft Stops)' '#SF018A_174' 'true' 'REQ: SF018A_174' '' } %GIDa_8fd82109_cb02_485f_8d12_8a304739c449
  Unary Minus : UnaryMinus  RequirementInfo={'linktype_rmi_doors' '0000ba56 (/E-STEER Core/SubSystem Specifications/Application Functions/SF018A End-of-Travel Actuator Management- EOT Impact and Soft Stops)' '#SF018A_169' 'true' 'REQ: SF018A_169' '' } %GIDa_4fe2e4a8_4c68_45aa_b0d2_9cbf7d4d750e
  Unary Minus1 : UnaryMinus  RequirementInfo={'linktype_rmi_doors' '0000ba56 (/E-STEER Core/SubSystem Specifications/Application Functions/SF018A End-of-Travel Actuator Management- EOT Impact and Soft Stops)' '#SF018A_169' 'true' 'REQ: SF018A_169' '' } %GIDa_acc654d3_89e5_4926_8237_06b050259ea7
  Unary Minus2 : UnaryMinus  RequirementInfo={'linktype_rmi_doors' '0000ba56 (/E-STEER Core/SubSystem Specifications/Application Functions/SF018A End-of-Travel Actuator Management- EOT Impact and Soft Stops)' '#SF018A_169' 'true' 'REQ: SF018A_169' '' } %GIDa_744fe6ce_adcf_44c3_9c49_540e5f0c8457
  LimPosn : Outport
  wires:
  Merge1/1 -> Subtract1/2
  Unary Minus2/1 -> If Action Subsystem3/1(In1)
  Unary Minus1/1 -> Relational Operator3/2
  Unary Minus/1 -> Relational Operator2/2
  Constant5/1 -> Unary Minus2/1
  Merge/1 -> Subtract/1
  Merge2/1 -> LimPosn/1, Data Store Write1/1
  Subtract1/1 -> If Action Subsystem4/1(In1)
  Subtract/1 -> If Action Subsystem5/1(In1)
  HwPosn/1 -> If2/1
  If2/1 -> If Action Subsystem5/Action
  If2/2 -> If Action Subsystem4/Action
  If Action Subsystem4/1(Out1) -> Merge2/2
  If Action Subsystem5/1(Out1) -> Merge2/1
  Constant4/1 -> Unary Minus1/1
  Constant3/1 -> Unary Minus/1
  [EotCcw] -> If Action Subsystem2/1(In1)
  Logical Operator1/1 -> If1/1
  If1/1 -> If Action Subsystem3/Action
  If1/2 -> If Action Subsystem2/Action
  If Action Subsystem2/1(Out1) -> Merge1/2
  If Action Subsystem3/1(Out1) -> Merge1/1
  Relational Operator3/1 -> Logical Operator1/2
  [EotCcw] -> Relational Operator3/1
  [EotCcw] -> Relational Operator2/1
  Relational Operator2/1 -> Logical Operator1/1
  [EotCw] -> If Action Subsystem/1(In1)
  Constant2/1 -> If Action Subsystem1/1(In1)
  Logical Operator/1 -> If/1
  If/1 -> If Action Subsystem1/Action
  If/2 -> If Action Subsystem/Action
  If Action Subsystem/1(Out1) -> Merge/2
  If Action Subsystem1/1(Out1) -> Merge/1
  Relational Operator1/1 -> Logical Operator/2
  Constant1/1 -> Relational Operator1/2
  [EotCw] -> Relational Operator1/1
  Constant/1 -> Relational Operator/2
  [EotCw] -> Relational Operator/1
  Relational Operator/1 -> Logical Operator/1
  EotCw/1 -> [EotCw]
  EotCcw/1 -> [EotCcw]
  RackTrvlLimrRngEna/1 -> [RackTrvlLimrRngEna]
  [RackTrvlLimrRngEna] -> If3/1
  If3/1 -> If Action Subsystem6/Action
  If3/2 -> If Action Subsystem7/Action
  If Action Subsystem6/1(Out1) -> Merge3/1
  If Action Subsystem7/1(Out1) -> Merge3/2
  Merge3/1 -> Subtract1/1, Subtract/2
  Constant6/1 -> If Action Subsystem6/1(In1)
  Constant8/1 -> If Action Subsystem7/1(In1)
